simulink model "CrazyflieSimulationPID_20ablock2"  (R2024b)
settings: Solver=VariableStepAuto  StartTime=0.0  StopTime=T  RelTol=1e-3
values from neighbouring files (symbols this model uses):
  noiseonppt = 0    [CrazyflieSimulationParameters.m]
  noiseonxyz = 0    [CrazyflieSimulationParameters.m]
  Ts = 1/100    (= 0.01)    [CrazyP2P.m]    (also in Drone4into12.m; ILCLinear.m; Tuning_script.m; p2p.m)
libraries: slpidlib x12, dspfdesign x6, simulink x6
(part 2 of 2)

== matlab function CrazyflieSimulationPID_20ablock2/Subsystem/2D Transform. - Refs ==
  data: x_I input; x_B output; y_I input; y_B output; psi_I input
function [x_B,y_B] = fcn(x_I,y_I,psi_I)

x_B =  cos(psi_I) * x_I + sin(psi_I) * y_I;
y_B = -sin(psi_I) * x_I + cos(psi_I) * y_I;

end

== matlab function CrazyflieSimulationPID_20ablock2/Subsystem/Angle Wrap-phi ==
  data: x input; y output
function y = wrapToPi(x)
    y = mod(x + pi, 2*pi) - pi;

== matlab function CrazyflieSimulationPID_20ablock2/Subsystem/3D Transformation ==
  data: u input; xd output; v input; yd output; w input; phi input; theta input; psi input; zd output
function [xd,yd,zd] = fcn(u,v,w,phi,theta,psi)

xd = w*(sin(psi)*sin(phi) + cos(psi)*cos(phi)*sin(theta)) - v*(sin(psi)*cos(phi) - cos(psi)*sin(phi)*sin(theta)) +u*cos(psi)*cos(theta);
yd = v*(cos(psi)*cos(phi) + sin(psi)*sin(phi)*sin(theta)) - w*(cos(psi)*sin(phi) - sin(psi)*cos(phi)*sin(theta)) +u*sin(psi)*cos(theta);
zd = w*(cos(psi)*cos(phi)) - u*sin(theta) + v*sin(phi)*cos(theta);

end

== matlab function CrazyflieSimulationPID_20ablock2/Subsystem/Quadcopter dynamic model ==
  data: U1 input; ud output; U2 input; U3 input; U4 input; phi input; p input; theta input; q input; psi input; r input; vd output; wd output; pd output; qd output; rd output; u input; v input; w input
function [ud,vd,wd,pd,qd,rd] = fcn(U1,U2,U3,U4,phi,p,theta,q,psi,r,u,v,w)

m = 0.028;                   % Mass (kg)
jxx = 16.571e-6;             % Moment of inertia around x-axis (kg·m²)
jyy = 16.656e-6;             % Moment of inertia around y-axis (kg·m²)
jzz = 29.262e-6;             % Moment of inertia around z-axis (kg·m²)
g = 9.81;                    % Acceleration due to gravity (m/s²)
 
ud = r*v - q*w + g*sin(theta);
vd = p*w - r*u - g*sin(phi)*cos(theta);
wd = q*u - p*v + U1/m - g*cos(theta)*cos(phi);

pd = ( -(jzz - jyy)*q*r + U2 ) / jxx;
qd = ( -(jxx - jzz)*p*r + U3 ) / jyy;
rd = ( -(jyy - jxx)*p*q + U4 ) / jzz;

end

== matlab function CrazyflieSimulationPID_20ablock2/Subsystem/Position Control ==
  data: u input; x_d output; y_d output; z_d output; psi_d output
function [x_d,y_d,z_d,psi_d] = fcn(u)
    %mine
    x_d = 1 - cos(2 * u);
    y_d = sin(2 * u);
    z_d = 2 * u;
    psi_d = 0*u;

%%%%%%%%%%%% OG %%%%%%%%%%%
    %x_d = 0.5*(1-cos(2*u));%1;
    %y_d = 0.5*sin(2*u);%1;
    %z_d = 0.1*u;%-5*9.81*u^2;
    %psi_d = 0;
end

== matlab function CrazyflieSimulationPID_20ablock2/Subsystem/2D Transform. - Actual ==
  data: x_I input; x_B output; y_I input; y_B output; psi_I input
function [x_B,y_B] = fcn(x_I,y_I,psi_I)

x_B =  cos(psi_I) * x_I + sin(psi_I) * y_I;
y_B = -sin(psi_I) * x_I + cos(psi_I) * y_I;

end

== matlab function CrazyflieSimulationPID_20ablock2/Subsystem/Angle Transformation ==
  data: p input; phid output; q input; r input; phi input; theta input; thetad output; psid output
function [phid,thetad,psid] = fcn(p,q,r,phi,theta)

phid   = p + q*sin(phi)*tan(theta) + r*cos(phi)*tan(theta);
thetad = q*cos(phi) - r*sin(phi);
psid   = q*sin(phi)/cos(theta) + r*cos(phi)/cos(theta);

== matlab function CrazyflieSimulationPID_20ablock2/Subsystem/Angle Wrap-psi ==
  data: x input; y output
function y = wrapToPi(x)
    y = mod(x + pi, 2*pi) - pi;
